simulink model "Auto_microgrid_forecasting_021622"  (R2020a)
settings: Solver=VariableStepAuto  StartTime=0.0  StopTime=50  MaxStep=1e-4  RelTol=1e-3
PreLoadFcn:
  | %run('FC_microgrid_param.m')
  | %load('gen_grid_init.mat')
InitFcn:
  | %load myisoModel_init;
  | run('FC_microgrid_param.m')
  | tic
  | run('CARTinitFcn.m')
  | %caseNo = 2;
  | 
  | %if (caseNo == 1)
  | %set_param(['Isolated_grid_paper_model_022521/SignalGen'], 'ActiveScenario', 'PStep222kW');
  | %else
  | %set_param(['Isolated_grid_paper_model_022521/SignalGen'], 'ActiveScenario', 'QStep222kVAr');
  | 
  | %end;
StopFcn:
  | toc
undefined symbols (not defined in the file or in its folder): breakpoints1, breakpoints2, cc_kp, cp_table_data, ctrl, D1, Delta, DiscIntNeverNeededParam, DT, FC_BESS, FC_PV_FirstSolar, find_system, Fnom, gcbh, libFC_BESS, libFC_PV, LowerLimit, magnitude, oversize, pll_ki, pll_kp, pq_ts, SOC_target, sps_rtmsupport, timer, Ts, ts, Ts_APC, Ts_Control, Ts_Power, UpperLimit
libraries: powerlib x151, simulink x100, powerlib_extras x100, powerlib_meascontrol x91, eePowerMeasurement x26, pi_ctrl x16, simulink_extras x12, sps_avr x7, eeGeneralControl x5, spsDieselMotorModel x3, libFSArray x2, SignalEditorBlockLib x2
(part 7 of 14)

== system Auto_microgrid_forecasting_021622/Grid Feeder Protective Relay/CS Modified PLL1/VCO ==
  w : Inport
  Compare To Constant : simulink/Logic and Bit Operations/Compare To Constant  relop=>=  const=pi  OutDataTypeStr=uint8
  Gain : Gain  Gain=2*pi  OutDataTypeStr=double
  Gain2 : Gain  Gain=Ts  SaturateOnIntegerOverflow=on  OutDataTypeStr=Inherit: Same as input  ParamDataTypeStr=Inherit: Same as input
  Sum : Sum  Inputs=-++
  Unit Delay1 : UnitDelay  SampleTime=-1  HasFrameUpgradeWarning=on
  theta : Outport
  wires:
  w/1 -> Gain2/1
  Gain/1 -> Sum/1
  Compare To Constant/1 -> Gain/1
  Unit Delay1/1 -> Compare To Constant/1, Sum/3, theta/1  "wt"
  Gain2/1 -> Sum/2
  Sum/1 -> Unit Delay1/1

== system Auto_microgrid_forecasting_021622/Grid Feeder Protective Relay/R25 - Sync Check v0.1/Freq_Comparator ==
  note: This block compares the frequency at the circuit breaker terminals
      | * if the difference is less than threshold dF_threshold, then outputs 1
  f_grid : Inport
  f_gen : Inport  Port=2
  dF_threshold : Inport  Port=3
  Fcn2 : Fcn  Expr=abs(u(2)-u(1)) <= u(3)
  Mux1 : Mux  Inputs=3
  Sum : Sum  Inputs=+-
  Locked : Outport
  dF : Outport  Port=2
  wires:
  Sum/1 -> dF/1
  f_grid/1 -> Mux1/1, Sum/2
  f_gen/1 -> Mux1/2, Sum/1
  dF_threshold/1 -> Mux1/3
  Fcn2/1 -> Locked/1
  Mux1/1 -> Fcn2/1

== system Auto_microgrid_forecasting_021622/Grid Feeder Protective Relay/R25 - Sync Check v0.1/Phase_Comparator ==
  note: This block compares the angle (phase A only) at the circuit breaker terminals
      | * if the difference is less than threshold angle_threshold, then outputs 1
  wt_grid : Inport
  wt_gen : Inport  Port=2
  angle_threshold : Inport  Port=3
  Abs : Abs
  Fcn1 : Fcn  Expr=u(1) <= u(2)  SampleTime=Ts
  Mux1 : Mux  Inputs=2
  Radians to Degrees : simulink_extras/Transformations/Radians to Degrees
  Scope : Scope
  Sum1 : Sum  Inputs=|-+
  WrapPi : Subsystem
  Locked : Outport
  dWt : Outport  Port=2
  wires:
  WrapPi/1(Out1) -> Abs/1, dWt/1
  Sum1/1 -> WrapPi/1(In1)
  wt_grid/1 -> Sum1/1
  wt_gen/1 -> Sum1/2
  Radians to Degrees/1 -> Scope/1, Mux1/1  "R2D"
  Mux1/1 -> Fcn1/1
  angle_threshold/1 -> Mux1/2
  Fcn1/1 -> Locked/1  "bool"
  Abs/1 -> Radians to Degrees/1  "diff"

== system Auto_microgrid_forecasting_021622/Grid Feeder Protective Relay/R25 - Sync Check v0.1/Voltage_Comparator ==
  note: This block compares the voltage at the circuit breaker terminals
      | * if the difference is less than threshold, then outputs 1
  note: dV_threshold% of the nominal VRMSLL
  V_bus : Inport
  V_line : Inport  Port=2
  dV_threshold : Inport  Port=3
  Fcn2 : Fcn  Expr=abs(u(2)-u(1)) <= u(3)
  Mux1 : Mux  Inputs=3
  Sum : Sum  Inputs=+-
  Locked : Outport
  dV : Outport  Port=2
  wires:
  Sum/1 -> dV/1
  dV_threshold/1 -> Mux1/3  "[%]"
  V_bus/1 -> Sum/2, Mux1/1
  V_line/1 -> Mux1/2, Sum/1
  Fcn2/1 -> Locked/1  "thshld"
  Mux1/1 -> Fcn2/1

== system Auto_microgrid_forecasting_021622/Grid Feeder Protective Relay1/CS Modified PLL/Controller ==
  note: Discrete PID Controller
  note: Pierre Giroux, Gilbert Sybille
      | Power System Simulation Laboratory
      | IREQ, Hydro-Quebc
  Error : Inport
  Discrete Derivative : simulink/Discrete/Discrete Derivative  gainval=1.0  ICPrevScaledInput=0.0  OutMin=[]  OutMax=[]  OutDataType=sfix(16)  OutScaling=2^-10  DoSatur=off
  Discrete-Time Integrator : DiscreteIntegrator  InitialCondition=Init  SampleTime=Ts  LimitOutput=on  UpperSaturationLimit=UpperLimit  LowerSaturationLimit=LowerLimit  ICPrevOutput=DiscIntNeverNeededParam  ICPrevScaledInput=DiscIntNeverNeededParam
  Kp4 : Gain  Gain=Kp  SaturateOnIntegerOverflow=on  OutDataTypeStr=Inherit: Same as input  ParamDataTypeStr=Inherit: Same as input
  Kp5 : Gain  Gain=Ki  SaturateOnIntegerOverflow=on  OutDataTypeStr=Inherit: Same as input  ParamDataTypeStr=Inherit: Same as input
  Kp6 : Gain  Gain=Kd  SaturateOnIntegerOverflow=on  OutDataTypeStr=Inherit: Same as input  ParamDataTypeStr=Inherit: Same as input
  Saturation2 : Saturate  UpperLimit=UpperLimit  LowerLimit=LowerLimit
  Sum6 : Sum  Inputs=+++  InputSameDT=on  SaturateOnIntegerOverflow=on  OutDataTypeStr=Inherit: Same as first input
  Zero-Order Hold : ZeroOrderHold  SampleTime=Ts
  Out : Outport  InitialOutput=0
  wires:
  Zero-Order Hold/1 -> Discrete Derivative/1
  Saturation2/1 -> Out/1
  Discrete Derivative/1 -> Sum6/3
  Discrete-Time Integrator/1 -> Sum6/2
  Kp4/1 -> Sum6/1
  Kp6/1 -> Zero-Order Hold/1
  Kp5/1 -> Discrete-Time Integrator/1
  Sum6/1 -> Saturation2/1
  Error/1 -> Kp6/1, Kp5/1, Kp4/1

== system Auto_microgrid_forecasting_021622/Grid Feeder Protective Relay1/CS Modified PLL/VCO ==
  w : Inport
  Compare To Constant : simulink/Logic and Bit Operations/Compare To Constant  relop=>=  const=pi  OutDataTypeStr=uint8
  Gain : Gain  Gain=2*pi  OutDataTypeStr=double
  Gain2 : Gain  Gain=Ts  SaturateOnIntegerOverflow=on  OutDataTypeStr=Inherit: Same as input  ParamDataTypeStr=Inherit: Same as input
  Sum : Sum  Inputs=-++
  Unit Delay1 : UnitDelay  SampleTime=-1  HasFrameUpgradeWarning=on
  theta : Outport
  wires:
  Sum/1 -> Unit Delay1/1
  Gain2/1 -> Sum/2
  Unit Delay1/1 -> theta/1, Sum/3, Compare To Constant/1  "wt"
  Compare To Constant/1 -> Gain/1
  Gain/1 -> Sum/1
  w/1 -> Gain2/1

== system Auto_microgrid_forecasting_021622/Grid Feeder Protective Relay1/CS Modified PLL1/Controller ==
  note: Discrete PID Controller
  note: Pierre Giroux, Gilbert Sybille
      | Power System Simulation Laboratory
      | IREQ, Hydro-Quebc
  Error : Inport
  Discrete Derivative : simulink/Discrete/Discrete Derivative  gainval=1.0  ICPrevScaledInput=0.0  OutMin=[]  OutMax=[]  OutDataType=sfix(16)  OutScaling=2^-10  DoSatur=off
  Discrete-Time Integrator : DiscreteIntegrator  InitialCondition=Init  SampleTime=Ts  LimitOutput=on  UpperSaturationLimit=UpperLimit  LowerSaturationLimit=LowerLimit  ICPrevOutput=DiscIntNeverNeededParam  ICPrevScaledInput=DiscIntNeverNeededParam
  Kp4 : Gain  Gain=Kp  SaturateOnIntegerOverflow=on  OutDataTypeStr=Inherit: Same as input  ParamDataTypeStr=Inherit: Same as input
  Kp5 : Gain  Gain=Ki  SaturateOnIntegerOverflow=on  OutDataTypeStr=Inherit: Same as input  ParamDataTypeStr=Inherit: Same as input
  Kp6 : Gain  Gain=Kd  SaturateOnIntegerOverflow=on  OutDataTypeStr=Inherit: Same as input  ParamDataTypeStr=Inherit: Same as input
  Saturation2 : Saturate  UpperLimit=UpperLimit  LowerLimit=LowerLimit
  Sum6 : Sum  Inputs=+++  InputSameDT=on  SaturateOnIntegerOverflow=on  OutDataTypeStr=Inherit: Same as first input
  Zero-Order Hold : ZeroOrderHold  SampleTime=Ts
  Out : Outport  InitialOutput=0
  wires:
  Zero-Order Hold/1 -> Discrete Derivative/1
  Saturation2/1 -> Out/1
  Discrete Derivative/1 -> Sum6/3
  Discrete-Time Integrator/1 -> Sum6/2
  Kp4/1 -> Sum6/1
  Kp6/1 -> Zero-Order Hold/1
  Kp5/1 -> Discrete-Time Integrator/1
  Sum6/1 -> Saturation2/1
  Error/1 -> Kp6/1, Kp5/1, Kp4/1

== system Auto_microgrid_forecasting_021622/Grid Feeder Protective Relay1/CS Modified PLL1/VCO ==
  w : Inport
  Compare To Constant : simulink/Logic and Bit Operations/Compare To Constant  relop=>=  const=pi  OutDataTypeStr=uint8
  Gain : Gain  Gain=2*pi  OutDataTypeStr=double
  Gain2 : Gain  Gain=Ts  SaturateOnIntegerOverflow=on  OutDataTypeStr=Inherit: Same as input  ParamDataTypeStr=Inherit: Same as input
  Sum : Sum  Inputs=-++
  Unit Delay1 : UnitDelay  SampleTime=-1  HasFrameUpgradeWarning=on
  theta : Outport
  wires:
  Sum/1 -> Unit Delay1/1
  Gain2/1 -> Sum/2
  Unit Delay1/1 -> theta/1, Sum/3, Compare To Constant/1  "wt"
  Compare To Constant/1 -> Gain/1
  Gain/1 -> Sum/1
  w/1 -> Gain2/1

== system Auto_microgrid_forecasting_021622/Grid Feeder Protective Relay1/R25 - Sync Check v0.1/Freq_Comparator ==
  note: This block compares the frequency at the circuit breaker terminals
      | * if the difference is less than threshold dF_threshold, then outputs 1
  f_grid : Inport
  f_gen : Inport  Port=2
  dF_threshold : Inport  Port=3
  Fcn2 : Fcn  Expr=abs(u(2)-u(1)) <= u(3)
  Mux1 : Mux  Inputs=3
  Sum : Sum  Inputs=+-
  Locked : Outport
  dF : Outport  Port=2
  wires:
  Mux1/1 -> Fcn2/1
  Fcn2/1 -> Locked/1
  dF_threshold/1 -> Mux1/3
  f_gen/1 -> Sum/1, Mux1/2
  f_grid/1 -> Sum/2, Mux1/1
  Sum/1 -> dF/1

== system Auto_microgrid_forecasting_021622/Grid Feeder Protective Relay1/R25 - Sync Check v0.1/Phase_Comparator ==
  note: This block compares the angle (phase A only) at the circuit breaker terminals
      | * if the difference is less than threshold angle_threshold, then outputs 1
  wt_grid : Inport
  wt_gen : Inport  Port=2
  angle_threshold : Inport  Port=3
  Abs : Abs
  Fcn1 : Fcn  Expr=u(1) <= u(2)  SampleTime=Ts
  Mux1 : Mux  Inputs=2
  Radians to Degrees : simulink_extras/Transformations/Radians to Degrees
  Scope : Scope
  Sum1 : Sum  Inputs=|-+
  WrapPi : Subsystem
  Locked : Outport
  dWt : Outport  Port=2
  wires:
  Abs/1 -> Radians to Degrees/1  "diff"
  Fcn1/1 -> Locked/1  "bool"
  angle_threshold/1 -> Mux1/2
  Mux1/1 -> Fcn1/1
  Radians to Degrees/1 -> Scope/1, Mux1/1  "R2D"
  wt_gen/1 -> Sum1/2
  wt_grid/1 -> Sum1/1
  Sum1/1 -> WrapPi/1(In1)
  WrapPi/1(Out1) -> dWt/1, Abs/1

== system Auto_microgrid_forecasting_021622/Grid Feeder Protective Relay1/R25 - Sync Check v0.1/Voltage_Comparator ==
  note: dV_threshold% of the nominal VRMSLL
  note: This block compares the voltage at the circuit breaker terminals
      | * if the difference is less than threshold, then outputs 1
  V_bus : Inport
  V_line : Inport  Port=2
  dV_threshold : Inport  Port=3
  Fcn2 : Fcn  Expr=abs(u(2)-u(1)) <= u(3)
  Mux1 : Mux  Inputs=3
  Sum : Sum  Inputs=+-
  Locked : Outport
  dV : Outport  Port=2
  wires:
  Mux1/1 -> Fcn2/1
  Fcn2/1 -> Locked/1  "thshld"
  V_line/1 -> Sum/1, Mux1/2
  V_bus/1 -> Mux1/1, Sum/2
  dV_threshold/1 -> Mux1/3  "[%]"
  Sum/1 -> dV/1

== system Auto_microgrid_forecasting_021622/MODEL STABILIZER/AllStringInverters/BESS Inverter ==
  ctrl : Inport
  Controlled Voltage Source : powerlib/Electrical Sources/Controlled Voltage Source  Initialize=on  Source_Type=AC  Amplitude=0  Phase=0  Frequency=0  Measurements=None
  Controlled Voltage Source1 : powerlib/Electrical Sources/Controlled Voltage Source  Initialize=on  Source_Type=AC  Amplitude=0  Phase=0  Frequency=0  Measurements=None
  Controlled Voltage Source2 : powerlib/Electrical Sources/Controlled Voltage Source  Initialize=on  Source_Type=AC  Amplitude=0  Phase=0  Frequency=0  Measurements=None
  Demux : Demux  Outputs=3
  A : PMIOPort  Side=Right
  N : PMIOPort  Port=2  Side=Left
  B : PMIOPort  Port=3  Side=Right
  C : PMIOPort  Port=4  Side=Right
  wires:
  Demux/1 -> Controlled Voltage Source/1
  Demux/2 -> Controlled Voltage Source1/1
  Demux/3 -> Controlled Voltage Source2/1
  ctrl/1 -> Demux/1
  connections:
  A/RConn1 -- Controlled Voltage Source/RConn1
  Controlled Voltage Source2/LConn1 -- Controlled Voltage Source/LConn1 -- Controlled Voltage Source1/LConn1 -- N/RConn1
  Controlled Voltage Source1/RConn1 -- B/RConn1
  Controlled Voltage Source2/RConn1 -- C/RConn1

== system Auto_microgrid_forecasting_021622/MODEL STABILIZER/AllStringInverters/Stab_control ==
  Uabc : Inport
  Uabc_inv : Inport  Port=2
  Iabc : Inport  Port=3
  CB_status : Inport  Port=4
  Control : Inport  Port=5
  Bus Creator1 : BusCreator  Inputs=2
  Bus Creator5 : BusCreator  Inputs=1
  Bus Selector : BusSelector  OutputSignals=p_ref,q_ref,f_ref,v_ref,GF_mode
  InvControl : Subsystem  mask{Ts=Ts_Control, Unpp=600, Pn=200e3}
      mask prompts: Ts "Control sample time [s]"; Unpp "Nominal AC voltage [Vpp]"; Pn "Nominal Power [W]"
      mask init:
      | Unom = Unpp / sqrt(3);
      | Inom = Pn/3/Unom;
  Rate Transition{,1..2,4..7,9..10} (9 alike) : RateTransition  Integrity=off  OutPortSampleTime=Ts_Control
  Rate Transition3 : RateTransition  OutPortSampleTime=Ts
  Rate Transition8 : RateTransition  OutPortSampleTime=Ts
  Step1 : Step  Time=99  SampleTime=0
  Step2 : Step  Time=100  After=-1  SampleTime=0
  Sum : Sum  Inputs=|++
  CtrlOut : Outport
  wires:
  Sum/1 -> Rate Transition8/1
  Rate Transition10/1 -> InvControl/2(Uabc_inv)
  Uabc_inv/1 -> Rate Transition10/1
  Control/1 -> Bus Selector/1
  Rate Transition6/1 -> InvControl/7(fref)
  Rate Transition5/1 -> InvControl/6(qref)
  Rate Transition7/1 -> InvControl/8(vref)
  Rate Transition9/1 -> InvControl/9(GF_mode_en)
  Bus Selector/5 -> Rate Transition9/1  "<GF_mode>"
  Bus Selector/4 -> Rate Transition7/1  "<v_ref>"
  Bus Selector/3 -> Rate Transition6/1  "<f_ref>"
  Bus Selector/2 -> Rate Transition5/1  "<q_ref>"
  Bus Selector/1 -> Rate Transition4/1  "<p_ref>"
  Bus Creator1/1 -> CtrlOut/1
  Bus Creator5/1 -> Bus Creator1/2  "ToCB"
  CB_status/1 -> Rate Transition2/1
  Uabc/1 -> Rate Transition/1
  Rate Transition3/1 -> Bus Creator1/1  "Uabc"
  InvControl/1(Uabc_ref) -> Rate Transition3/1
  Rate Transition8/1 -> Bus Creator5/1  "Close"
  Rate Transition/1 -> InvControl/1(Uabc)
  Rate Transition1/1 -> InvControl/3(Iabc)
  Rate Transition2/1 -> InvControl/4(cb_stat)
  Iabc/1 -> Rate Transition1/1
  Rate Transition4/1 -> InvControl/5(pref)
  Step1/1 -> Sum/1
  Step2/1 -> Sum/2

== system Auto_microgrid_forecasting_021622/MODEL STABILIZER/AllStringInverters/Subsystem1 ==
  SmaINV : powerlib/Measurements/Three-Phase V-I Measurement  VoltageMeasurement=phase-to-ground  SetLabelV=off  LabelV=circuit_Usmainv  Vpu=off  VpuLL=off  CurrentMeasurement=yes  SetLabelI=off  LabelI=circuit_Ismainv  Ipu=off  Pbase=100e6  Vbase=500e3  OutputType=Complex  PhasorSimulation=off  PSBequivalent=0
  A : PMIOPort  Side=Left
  a : PMIOPort  Port=2  Side=Right
  B : PMIOPort  Port=3  Side=Left
  b : PMIOPort  Port=4  Side=Right
  C : PMIOPort  Port=5  Side=Left
  c : PMIOPort  Port=6  Side=Right
  tag scope: Iinv=scoped, Uinv=scoped
  wires:
  SmaINV/1 -> [Uinv]
  SmaINV/2 -> [Iinv]
  connections:
  SmaINV/RConn1 -- a/RConn1
  C/RConn1 -- SmaINV/LConn3
  SmaINV/LConn2 -- B/RConn1
  SmaINV/RConn2 -- b/RConn1
  SmaINV/RConn3 -- c/RConn1
  A/RConn1 -- SmaINV/LConn1

== system Auto_microgrid_forecasting_021622/MODEL STABILIZER/AllStringInverters/Subsystem2 ==
  GRI1 : powerlib/Measurements/Three-Phase V-I Measurement  VoltageMeasurement=phase-to-ground  SetLabelV=off  LabelV=Ugri  Vpu=off  VpuLL=off  CurrentMeasurement=yes  SetLabelI=off  LabelI=Igri  Ipu=off  Pbase=100e6  Vbase=500e3  OutputType=Complex  PhasorSimulation=off  PSBequivalent=0
  A : PMIOPort  Side=Left
  B : PMIOPort  Port=2  Side=Left
  a : PMIOPort  Port=3  Side=Right
  b : PMIOPort  Port=4  Side=Right
  C : PMIOPort  Port=5  Side=Left
  c : PMIOPort  Port=6  Side=Right
  tag scope: Igri=scoped, Ugri=scoped
  wires:
  GRI1/1 -> [Ugri]
  GRI1/2 -> [Igri]
  connections:
  GRI1/LConn3 -- C/RConn1
  GRI1/LConn2 -- B/RConn1
  GRI1/RConn3 -- c/RConn1
  GRI1/RConn2 -- b/RConn1
  GRI1/LConn1 -- A/RConn1
  GRI1/RConn1 -- a/RConn1

== system Auto_microgrid_forecasting_021622/Stab1/AllStringInverters/BESS Inverter ==
  ctrl : Inport
  Controlled Voltage Source : powerlib/Electrical Sources/Controlled Voltage Source  Initialize=on  Source_Type=AC  Amplitude=0  Phase=0  Frequency=0  Measurements=None
  Controlled Voltage Source1 : powerlib/Electrical Sources/Controlled Voltage Source  Initialize=on  Source_Type=AC  Amplitude=0  Phase=0  Frequency=0  Measurements=None
  Controlled Voltage Source2 : powerlib/Electrical Sources/Controlled Voltage Source  Initialize=on  Source_Type=AC  Amplitude=0  Phase=0  Frequency=0  Measurements=None
  Demux : Demux  Outputs=3
  A : PMIOPort  Side=Right
  N : PMIOPort  Port=2  Side=Left
  B : PMIOPort  Port=3  Side=Right
  C : PMIOPort  Port=4  Side=Right
  wires:
  ctrl/1 -> Demux/1
  Demux/3 -> Controlled Voltage Source2/1
  Demux/2 -> Controlled Voltage Source1/1
  Demux/1 -> Controlled Voltage Source/1
  connections:
  Controlled Voltage Source2/RConn1 -- C/RConn1
  Controlled Voltage Source1/RConn1 -- B/RConn1
  N/RConn1 -- Controlled Voltage Source1/LConn1 -- Controlled Voltage Source/LConn1 -- Controlled Voltage Source2/LConn1
  A/RConn1 -- Controlled Voltage Source/RConn1

== system Auto_microgrid_forecasting_021622/Stab1/AllStringInverters/PV_Control ==
  Uabc : Inport
  Uabc_inv : Inport  Port=2
  Iabc : Inport  Port=3
  CB_status : Inport  Port=4
  Control : Inport  Port=5
  Bus Creator1 : BusCreator  Inputs=2
  Bus Creator5 : BusCreator  Inputs=1
  Bus Selector : BusSelector  OutputSignals=p_ref,q_ref,f_ref,v_ref,GF_mode
  InvControl : Subsystem  mask{Ts=Ts_Control, Unpp=600, Pn=430e3}
      mask prompts: Ts "Control sample time [s]"; Unpp "Nominal AC voltage [Vpp]"; Pn "Nominal Power [W]"
      mask init:
      | Unom = Unpp / sqrt(3);
      | Inom = Pn/3/Unom;
  Rate Transition{,1..2,4..7,9..10} (9 alike) : RateTransition  Integrity=off  OutPortSampleTime=Ts_Control
  Rate Transition3 : RateTransition  OutPortSampleTime=Ts
  Rate Transition8 : RateTransition  OutPortSampleTime=Ts
  Step : Step  Time=3  SampleTime=0
  Step1 : Step  Time=6.4  SampleTime=0
  Sum : Sum  Inputs=|++
  CtrlOut : Outport
  wires:
  Step1/1 -> Sum/2
  Step/1 -> Sum/1
  Rate Transition4/1 -> InvControl/5(pref)
  Iabc/1 -> Rate Transition1/1
  Rate Transition2/1 -> InvControl/4(cb_stat)
  Rate Transition1/1 -> InvControl/3(Iabc)
  Rate Transition/1 -> InvControl/1(Uabc)
  Rate Transition8/1 -> Bus Creator5/1  "Close"
  Sum/1 -> Rate Transition8/1
  InvControl/1(Uabc_ref) -> Rate Transition3/1
  Rate Transition3/1 -> Bus Creator1/1  "Uabc"
  Uabc/1 -> Rate Transition/1
  CB_status/1 -> Rate Transition2/1
  Bus Creator5/1 -> Bus Creator1/2  "ToCB"
  Bus Creator1/1 -> CtrlOut/1
  Bus Selector/1 -> Rate Transition4/1  "<p_ref>"
  Bus Selector/2 -> Rate Transition5/1  "<q_ref>"
  Bus Selector/3 -> Rate Transition6/1  "<f_ref>"
  Bus Selector/4 -> Rate Transition7/1  "<v_ref>"
  Bus Selector/5 -> Rate Transition9/1  "<GF_mode>"
  Rate Transition9/1 -> InvControl/9(GF_mode_en)
  Rate Transition7/1 -> InvControl/8(vref)
  Rate Transition5/1 -> InvControl/6(qref)
  Rate Transition6/1 -> InvControl/7(fref)
  Control/1 -> Bus Selector/1
  Uabc_inv/1 -> Rate Transition10/1
  Rate Transition10/1 -> InvControl/2(Uabc_inv)

== system Auto_microgrid_forecasting_021622/Stab1/AllStringInverters/Subsystem1 ==
  SmaINV : powerlib/Measurements/Three-Phase V-I Measurement  VoltageMeasurement=phase-to-ground  SetLabelV=off  LabelV=circuit_Usmainv  Vpu=off  VpuLL=off  CurrentMeasurement=yes  SetLabelI=off  LabelI=circuit_Ismainv  Ipu=off  Pbase=100e6  Vbase=500e3  OutputType=Complex  PhasorSimulation=off  PSBequivalent=0
  A : PMIOPort  Side=Left
  a : PMIOPort  Port=2  Side=Right
  B : PMIOPort  Port=3  Side=Left
  b : PMIOPort  Port=4  Side=Right
  C : PMIOPort  Port=5  Side=Left
  c : PMIOPort  Port=6  Side=Right
  tag scope: Iinv=scoped, Uinv=scoped
  wires:
  SmaINV/2 -> [Iinv]
  SmaINV/1 -> [Uinv]
  connections:
  A/RConn1 -- SmaINV/LConn1
  SmaINV/RConn3 -- c/RConn1
  SmaINV/RConn2 -- b/RConn1
  SmaINV/LConn2 -- B/RConn1
  C/RConn1 -- SmaINV/LConn3
  SmaINV/RConn1 -- a/RConn1

== system Auto_microgrid_forecasting_021622/Stab1/AllStringInverters/Subsystem2 ==
  GRI1 : powerlib/Measurements/Three-Phase V-I Measurement  VoltageMeasurement=phase-to-ground  SetLabelV=off  LabelV=Ugri  Vpu=off  VpuLL=off  CurrentMeasurement=yes  SetLabelI=off  LabelI=Igri  Ipu=off  Pbase=100e6  Vbase=500e3  OutputType=Complex  PhasorSimulation=off  PSBequivalent=0
  A : PMIOPort  Side=Left
  B : PMIOPort  Port=2  Side=Left
  a : PMIOPort  Port=3  Side=Right
  b : PMIOPort  Port=4  Side=Right
  C : PMIOPort  Port=5  Side=Left
  c : PMIOPort  Port=6  Side=Right
  tag scope: Igri=scoped, Ugri=scoped
  wires:
  GRI1/2 -> [Igri]
  GRI1/1 -> [Ugri]
  connections:
  GRI1/RConn1 -- a/RConn1
  GRI1/LConn1 -- A/RConn1
  GRI1/RConn2 -- b/RConn1
  GRI1/RConn3 -- c/RConn1
  GRI1/LConn2 -- B/RConn1
  GRI1/LConn3 -- C/RConn1

== system Auto_microgrid_forecasting_021622/Wind Turbine Type 4/APC (atomic)1/Baseline ==
  Action Port : ActionPort  ActionPortLabel=case [ 5 ]:
  Constant1 : Constant  Value=0
  Qcmd : Outport
  dP : Outport  Port=2
  dT : Outport  Port=3
  wires:
  Constant1/1 -> dP/1, dT/1, Qcmd/1

== system Auto_microgrid_forecasting_021622/Wind Turbine Type 4/APC (atomic)1/Inertial Response (to df) ==
  Freq (Hz) : Inport
  type1 : Inport  Port=2
  wg (pu) : Inport  Port=3
  f_setpoint : Inport  Port=4
  Action Port : ActionPort  ActionPortLabel=case [ 1 ]:
  Constant1 : Constant  Value=0
  Constant2 : Constant  Value=0
  Constant3 : Constant  Value=1e-3
  Display{3..4,6..7} (4 alike) : Display
  Divide1 : Product  Inputs=*/
  FBIC : Subsystem
  Gain : Gain  Gain=Fnom
  Lock2 : Subsystem
  Rate Limiter1 : RateLimiter  RisingSlewLimit=0.45  SampleTimeMode=inherited
  Relational Operator3 : RelationalOperator  OutDataTypeStr=boolean  RndMeth=Nearest
  Relational Operator4 : RelationalOperator  Operator=<=  OutDataTypeStr=boolean  RndMeth=Nearest
  Saturation : Saturate  UpperLimit=0.4  LowerLimit=0
  Saturation1 : Saturate  UpperLimit=1  LowerLimit=1e-5
  Scope : Scope  NumInputPorts=3
  Sum1 : Sum  Inputs=|-+
  Switch1 : Switch  Criteria=u2 > Threshold  Threshold=1
  TLIC : Subsystem  TreatAsAtomicUnit=on
  Type1 : Switch  Criteria=u2 > Threshold  Threshold=0.5
  When to start IR : DigitalClock  SampleTime=-1
  dead band1 : Constant  Value=0.2
  dT : Outport
  dP : Outport  Port=2
  Qcmd : Outport  Port=3
  wires:
  Constant1/1 -> dP/1, Qcmd/1
  Constant2/1 -> Switch1/3
  When to start IR/1 -> Switch1/2
  Lock2/1(O) -> Switch1/1
  Saturation/1 -> dT/1
  wg (pu)/1 -> [Wg], FBIC/1(wg (pu))
  Switch1/1 -> Display3/1, Scope/3, [In_Act]
  type1/1 -> Type1/2
  Sum1/1 -> Relational Operator3/1, Scope/2
  FBIC/1(Delta_P FBIC1) -> Type1/3
  Type1/1 -> [Delta_P], Display6/1
  Freq (Hz)/1 -> FBIC/2(Freq (Hz)1), [Freq]
  [In_Act] -> FBIC/3(Act1), TLIC/1(Act)
  TLIC/1(Delta_P TLIC) -> Type1/1
  [Delta_P] -> Relational Operator4/1
  f_setpoint/1 -> Gain/1
  dead band1/1 -> Relational Operator3/2
  Divide1/1 -> Rate Limiter1/1
  [Wg] -> Saturation1/1
  Saturation1/1 -> Divide1/2
  Constant3/1 -> Relational Operator4/2
  Relational Operator4/1 -> Display7/1, Lock2/2(R)
  [Freq] -> Sum1/1, Display4/1
  [Delta_P] -> Divide1/1, Scope/1
  Relational Operator3/1 -> Lock2/1(I)
  Rate Limiter1/1 -> Saturation/1
  Gain/1 -> Sum1/2

== system Auto_microgrid_forecasting_021622/Wind Turbine Type 4/APC (atomic)1/PFR ==
  Freq (Hz) : Inport
  f_setpoint : Inport  Port=2
  Action Port : ActionPort  ActionPortLabel=case [ 2 3 ]:
  Constant1 : Constant  Value=0
  Dead Zone : DeadZone  LowerValue=-db/60  UpperValue=db/60  SaturateOnIntegerOverflow=on
  Divide1 : Product  Inputs=*/
  Gain : Gain  Gain=Fnom
  P/f gain : Gain  Gain=1/k
  Saturation : Saturate  UpperLimit=0
  Sum : Sum  Inputs=|+-
  Sum1 : Sum  Inputs=|-+
  curtailment pu : Constant  Value=0.2
  dP : Outport
  dT : Outport  Port=2
  Qcmd : Outport  Port=3
  wires:
  Sum/1 -> Saturation/1
  Constant1/1 -> dT/1, Qcmd/1
  Saturation/1 -> dP/1
  P/f gain/1 -> Sum/1
  curtailment pu/1 -> Sum/2
  Dead Zone/1 -> P/f gain/1
  f_setpoint/1 -> Gain/1
  Freq (Hz)/1 -> Sum1/1
  Divide1/1 -> Dead Zone/1  "delta f pu"
  Sum1/1 -> Divide1/1
  Gain/1 -> Sum1/2, Divide1/2

== system Auto_microgrid_forecasting_021622/Wind Turbine Type 4/APC (atomic)1/PQ ==
  SFRcmd : Inport
  Qin : Inport  Port=2
  Action Port : ActionPort  ActionPortLabel=case [ 4 ]:
  Constant : Constant
  Constant1 : Constant  Value=0
  Sum : Sum  Inputs=|+-
  dP : Outport
  Qcmd : Outport  Port=2
  dT : Outport  Port=3
  wires:
  Constant1/1 -> dT/1
  Qin/1 -> Qcmd/1
  Constant/1 -> Sum/2
  Sum/1 -> dP/1
  SFRcmd/1 -> Sum/1

== system Auto_microgrid_forecasting_021622/Wind Turbine Type 4/Control/Excitation Control system ==
  Flux : Inport
  wr : Inport  Port=2
  Discrete PI Controller : Subsystem  DialogController=POWERSYS.PowerSysDialog  mask(Discrete PI Controller){Kp=Kp_field, Ki=Ki_field, Par_Limits=[1 0]*Vf_limit, Init=init(9), Ts=Ts}
      mask prompts: Kp "Proportional gain (Kp):"; Ki "Integral gain (Ki):"; Par_Limits "Output limits: [ Upper   Lower ]"; Init "Output initial value:"; Ts "Sample time:"
      mask help: This block implements a discrete PI controller.
      mask init:
      | UpperLimit=Par_Limits(1);
      | LowerLimit=Par_Limits(2);
      | power_initmask();
      mask Help: This block is part of a subset of blocks in the Extras library that does not have documentation associated with it, other than the block mask description.
      mask Display: disp('PI');
  Divide : Product  Inputs=*/
  Flux_ref : Constant
  "Flux_ref " : Constant
  Sum4 : Sum  Inputs=|+-  InputSameDT=on  SaturateOnIntegerOverflow=on  OutDataTypeStr=Inherit: Same as first input
  Switch : Switch  Threshold=1
  avoid division by 0 : Saturate  UpperLimit=inf  LowerLimit=1e-6
  Vf : Outport  VectorParamsAs1DForOutWhenUnconnected=off
  wires:
  Sum4/1 -> Discrete PI Controller/1(Error)
  Discrete PI Controller/1(Out) -> Vf/1  "Vf"
  Flux/1 -> Sum4/2  "Flux"
  wr/1 -> Switch/2, avoid division by 0/1
  Flux_ref/1 -> Switch/3
  "Flux_ref "/1 -> Divide/1
  avoid division by 0/1 -> Divide/2
  Divide/1 -> Switch/1
  Switch/1 -> Sum4/1

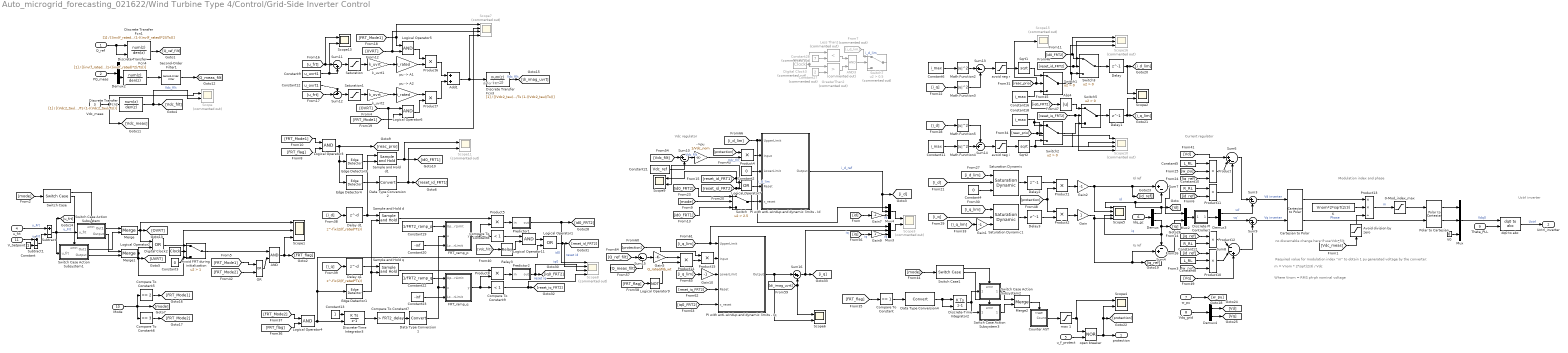
== system Auto_microgrid_forecasting_021622/Wind Turbine Type 4/Control/Grid-Side Inverter Control ==
  note: no discernable change here if use Vdc_filt
  note: di for FRT
  note: Required value for modulation index "m" to obtain 1 pu generated voltage by the converter:
  note: Modulation index and phase
  note: Where Vnom = RMS ph-ph nominal voltage
  note: Uctrl inverter
  note: Current regulator
  note: Iq ref
  note: m = Vnom * 2*sqrt(2/3) / Vdc
  note: Id ref
  note: Vdc regulator
  Q_ref : Inport
  PQ_meas : Inport  Port=2
  Vdc_meas : Inport  Port=3
  u_frt : Inport  Port=4
  u_f_protect : Inport  Port=5
  Idq_gc : Inport  Port=6
  w_pu : Inport  Port=7
  Vdq_grid : Inport  Port=8
  Theta_PLL : Inport  Port=9
  Mode : Inport  Port=10
  V_Setpoint : Inport  Port=11
  ->pu : Gain  Gain=1/Vdc_nom
  0-Mod_index_max : Saturate  UpperLimit=Mod_index_max  LowerLimit=0
  AND : Logic  IconShape=distinctive  AllPortsSameDT=off  OutDataTypeStr=boolean
  AND3 : Logic  Commented=on  IconShape=distinctive  AllPortsSameDT=off  OutDataTypeStr=boolean
  Abs4 : Abs
  Add1 : Sum
  Avoid FRT during initialization : Switch  Criteria=u2 > Threshold  Threshold=1
  Avoid division by zero : Saturate  UpperLimit=1e6  LowerLimit=1e-6
  Cartesian to Polar : simulink_extras/Transformations/Cartesian to Polar
  Compare To Constant : simulink/Logic and Bit Operations/Compare To Constant  relop===  const=1  OutDataTypeStr=boolean
  Compare To Constant5 : simulink/Logic and Bit Operations/Compare To Constant  relop===  const=2  OutDataTypeStr=boolean
  Compare To Constant6 : simulink/Logic and Bit Operations/Compare To Constant  relop===  const=3  OutDataTypeStr=boolean
  Compare To Constant7 : simulink/Logic and Bit Operations/Compare To Constant  relop=>  const=FRT2_delay  OutDataTypeStr=boolean
  Compare To Constant8 : simulink/Logic and Bit Operations/Compare To Constant  relop=<  const=1  OutDataTypeStr=boolean
  Compare To Constant9 : simulink/Logic and Bit Operations/Compare To Constant  relop=<  const=1  OutDataTypeStr=boolean
  Constant : Constant
  Constant10 : Constant  Value=R_RL
  Constant{6,11,16,18} (4 alike) : Constant  Value=i_max  SampleTime=Ts
  Constant12 : Constant  Value=u_ovrt1  SampleTime=Ts
  Constant13 : Constant
  Constant17 : Constant  Value=R_RL
  Constant19 : Constant  Value=1/FRT2_ramp_p  SampleTime=Ts
  Constant2 : Constant  Value=0  SampleTime=Ts
  Constant20 : Constant  Value=-inf  SampleTime=Ts
  Constant21 : Constant  Value=Vdc_ref  SampleTime=Ts
  Constant22 : Constant  Value=1/FRT2_ramp_q  SampleTime=Ts
  Constant23 : Constant  Value=-inf  SampleTime=Ts
  Constant27 : Constant  Commented=on  Value=2
  Constant28 : Constant  Commented=on  Value=7
  Constant3 : Constant  Value=0
  Constant4 : Constant  Value=0  SampleTime=Ts
  Constant5 : Constant  Value=L_RL
  Constant8 : Constant  Value=L_RL
  Constant9 : Constant  Value=u_uvrt1  SampleTime=Ts
  Counter AST : Subsystem
  Data Type Conversion1 : DataTypeConversion
  Data Type Conversion2 : DataTypeConversion
  Data Type Conversion4 : DataTypeConversion
  Delay{,1..3} (4 alike) : Delay  DelayLength=1  InitialCondition=0  SampleTime=Ts
  Delay d1 : Delay  DelayLength=fix(2/(f_rated*Ts))  InitialCondition=1  SampleTime=Ts
  Delay q1 : Delay  DelayLength=fix(2/(f_rated*Ts))  InitialCondition=1  SampleTime=Ts
  Demux{,2..4} (4 alike) : Demux  Outputs=2
      Demux settings: DisplayOption=none
      Demux3 settings: DisplayOption=none
      Demux4 settings: DisplayOption=none
  Digital Clock2 : DigitalClock  SampleTime=Ts
  Digital Clock3 : DigitalClock  Commented=on  SampleTime=-1
  Discrete PI Controller1 : Subsystem  DialogController=POWERSYS.PowerSysDialog  mask(Discrete PI Controller){Kp=Kp_grid_side_cur_reg, Ki=Ki_grid_side_cur_reg, Par_Limits=[1 -1]*Current_reg_output_limit, Init=0, Ts=Ts}
      mask prompts: Kp "Proportional gain (Kp):"; Ki "Integral gain (Ki):"; Par_Limits "Output limits: [ Upper   Lower ]"; Init "Output initial value:"; Ts "Sample time:"
      mask help: This block implements a discrete PI controller.
      mask init:
      | UpperLimit=Par_Limits(1);
      | LowerLimit=Par_Limits(2);
      | power_initmask();
      mask Help: This block is part of a subset of blocks in the Extras library that does not have documentation associated with it, other than the block mask description.
      mask Display: disp('PI');
  Discrete Transfer Fcn1 : DiscreteTransferFcn  Denominator=[(inv(f_rated)*2)/Ts (1-((inv(f_rated)*2)/Ts))]  InitialStatesSource=Input port  SampleTime=Ts
      settings: InputPortMap=u0,p5
  Discrete Transfer Fcn2 : DiscreteTransferFcn  Denominator=[(Vdc2_tau)/Ts (1-((Vdc2_tau)/Ts))]  InitialStates=Vdc2_filt_init  SampleTime=Ts
  Discrete Transfer Fcn3 : DiscreteTransferFcn  Denominator=[(Vdc2_tau)/Ts (1-((Vdc2_tau)/Ts))]  SampleTime=Ts
  Discrete Transfer Fcn4 : DiscreteTransferFcn  Denominator=[(inv(f_rated)*2)/Ts (1-((inv(f_rated)*2)/Ts))]  InitialStates=U_rated^2/(-inv(2*pi*f_rated*Cshunt_filter))  SampleTime=Ts
  Discrete-Time Integrator2 : DiscreteIntegrator  ExternalReset=falling  SampleTime=Ts  ICPrevOutput=DiscIntNeverNeededParam  ICPrevScaledInput=DiscIntNeverNeededParam
  Discrete-Time Integrator3 : DiscreteIntegrator  ExternalReset=level  SampleTime=Ts  LimitOutput=on  UpperSaturationLimit=1  LowerSaturationLimit=0  ICPrevOutput=DiscIntNeverNeededParam  ICPrevScaledInput=DiscIntNeverNeededParam
  Edge Detector1 : powerlib_meascontrol/Logic/Edge Detector  model=Rising  ic=0  Ts=Ts
      settings: SourceProductBaseCode=PS
  Edge Detector3 : powerlib_meascontrol/Logic/Edge Detector  model=Rising  ic=0  Ts=Ts
      settings: SourceProductBaseCode=PS
  Edge Detector4 : powerlib_meascontrol/Logic/Edge Detector  model=Falling  ic=0  Ts=Ts
      settings: SourceProductBaseCode=PS
  FRT_ramp_p : Subsystem
  FRT_ramp_q : Subsystem
  From7 : From  Commented=on  GotoTag=i_d_lim
  Gain : Gain
  Gain{1..2,7,10} (4 alike) : Gain  Gain=-1
  Gain5 : Gain  Gain=Q_rated/Nb_wt
  Gain9 : Gain
  GreaterThan2 : RelationalOperator  Commented=on  Operator=>  OutDataTypeStr=boolean  RndMeth=Simplest
  K : Constant  Value=Vnom*2*sqrt(2/3)
  Less Than2 : RelationalOperator  Commented=on  Operator=<  OutDataTypeStr=boolean  RndMeth=Simplest
  Logical Operator1 : Logic  Operator=OR  AllPortsSameDT=off  OutDataTypeStr=boolean
  Logical Operator{3..6,11} (5 alike) : Logic  AllPortsSameDT=off  OutDataTypeStr=boolean
  Logical Operator2 : Logic  Operator=OR  AllPortsSameDT=off  OutDataTypeStr=boolean
  Logical Operator7 : Logic  Operator=OR  AllPortsSameDT=off  OutDataTypeStr=boolean
  Logical Operator9 : Logic  Operator=NOT  AllPortsSameDT=off  OutDataTypeStr=boolean
  Math Function{2..5} (4 alike) : Math  Operator=magnitude^2  SignedPower=on  SaturateOnIntegerOverflow=on
  Merge : Merge
  Merge1 : Merge
  Merge2 : Merge
  Mux : Mux  Inputs=3
  Mux2 : Mux  Inputs=2
  Mux3 : Mux  Inputs=3
  Mux4 : Mux  Inputs=3
  OR : Logic  Operator=OR  IconShape=distinctive  AllPortsSameDT=off  OutDataTypeStr=boolean
  PI with anti-windup and dynamic limits - Id : Subsystem  mask(Discrete PI Controller with anti-windup and dynamic limiters){Kp=Kp_dc, Ki=Ki_dc, Init=Vdc_nom, Ts=Ts}
      mask prompts: Kp "Proportional gain (Kp):"; Ki "Integral gain (Ki):"; Init "State initial value:"; Ts "Sample time:"
      mask Display:
      | disp('PI-\nAST');
      | port_label('input',1,'Max');
      | port_label('input',2,'In');
      | port_label('input',3,'Min');
      | port_label('input',4,'Reset');
      | port_label('input',5,'x_reset');
      | port_label('output',1,'Out');
  PI with anti-windup and dynamic limits - Iq : Subsystem  mask(Discrete PI Controller with anti-windup and dynamic limiters){Kp=Q_Kp/1000, Ki=Q_Ki/1000, Init=0, Ts=Ts}
      mask prompts: Kp "Proportional gain (Kp):"; Ki "Integral gain (Ki):"; Init "State initial value:"; Ts "Sample time:"
      mask Display:
      | disp('PI-\nAST');
      | port_label('input',1,'Max');
      | port_label('input',2,'In');
      | port_label('input',3,'Min');
      | port_label('input',4,'Reset');
      | port_label('input',5,'x_reset');
      | port_label('output',1,'Out');
  Polar to Cartesian : simulink_extras/Transformations/Polar to Cartesian
      settings: SourceProductBaseCode=SL
  Predictor1 : Subsystem  mask{Init_value=0, Ts=Ts}
      mask prompts: Init_value "Initial value:"; Ts "Sample time (Ts):"
  Predictor2 : Subsystem  mask{Init_value=0, Ts=Ts}
      mask prompts: Init_value "Initial value:"; Ts "Sample time (Ts):"
  Product : Product  Inputs=3  InputSameDT=on  SaturateOnIntegerOverflow=on  OutDataTypeStr=Inherit: Same as first input
  Product{1..2,4..8,14..15} (9 alike) : Product
  Product10 : Product  Inputs=3  InputSameDT=on  SaturateOnIntegerOverflow=on  OutDataTypeStr=Inherit: Same as first input
  Product11 : Product  InputSameDT=on  SaturateOnIntegerOverflow=on  OutDataTypeStr=Inherit: Same as first input
  Product12 : Product  InputSameDT=on  SaturateOnIntegerOverflow=on  OutDataTypeStr=Inherit: Same as first input
  Product13 : Product  Inputs=**/  InputSameDT=on  SaturateOnIntegerOverflow=on  OutDataTypeStr=Inherit: Same as first input
  Relay3 : Relay  OnSwitchValue=1.02*Vdc_ref  OffSwitchValue=1.015*Vdc_ref  OutDataTypeStr=Inherit: Inherit via back propagation
  Sample and Hold d : powerlib_meascontrol/Additional Components/Sample and Hold  ic=0  Ts=Ts
      settings: SourceProductBaseCode=PS
  Sample and Hold d1 : powerlib_meascontrol/Additional Components/Sample and Hold  ic=0  Ts=Ts
      settings: SourceProductBaseCode=PS
  Sample and Hold q : powerlib_meascontrol/Additional Components/Sample and Hold  ic=0  Ts=Ts
      settings: SourceProductBaseCode=PS
  Saturation : Saturate  UpperLimit=0.08  LowerLimit=0
  Saturation Dynamic : simulink/Discontinuities/Saturation Dynamic  OutMin=[]  OutMax=[]  OutDataTypeStr=Inherit: Same as second input  OutDataType=fixdt(1, 16)  OutScaling=2^-10  DoSatur=off
  Saturation Dynamic1 : simulink/Discontinuities/Saturation Dynamic  OutMin=[]  OutMax=[]  OutDataTypeStr=Inherit: Same as second input  OutDataType=fixdt(1, 16)  OutScaling=2^-10  DoSatur=off
  Saturation1 : Saturate  UpperLimit=0  LowerLimit=-0.08
  Scope : Scope  Commented=on  NumInputPorts=2
  Scope1 : Scope  NumInputPorts=3
  Scope10 : Scope  Commented=on  NumInputPorts=4
  Scope11 : Scope  Commented=on  NumInputPorts=2
  Scope{2,4,6,9,13} (5 alike) : Scope  NumInputPorts=2
  Scope15 : Scope  Commented=on
  Scope16 : Scope  Commented=on  NumInputPorts=3
  Scope3 : Scope  Commented=on  NumInputPorts=2
  Scope5 : Scope  NumInputPorts=4
  Scope7 : Scope  Commented=on  NumInputPorts=4
  Scope8 : Scope  Commented=on  NumInputPorts=4
  Second-Order Filter1 : powerlib_meascontrol/Filters/Second-Order Filter  FilterType=Lowpass  Fo=Freq_filter  Zeta=Zeta_filter  Ts=Ts  Initialize=off  Vac_Init="[0,  0,  60]"  Vdc_Init=0  PlotResponse=off  FreqRange=[0, 500, 1]
      settings: SourceProductBaseCode=MT,PS
  Sqrt1 : Sqrt  SaturateOnIntegerOverflow=on
  Sqrt2 : Sqrt  SaturateOnIntegerOverflow=on
  Subtract : Sum  Inputs=+-
  Subtract1 : Sum  Inputs=+-
  Sum10 : Sum  Inputs=|+-
  Sum11 : Sum  Inputs=|-+
  Sum12 : Sum  Inputs=+-|
  Sum13 : Sum  Inputs=|+-
  Sum14 : Sum  Inputs=-+|
  Sum15 : Sum  Inputs=|+-
  Sum16 : Sum  Inputs=|++
  Sum3 : Sum  Inputs=|+-  InputSameDT=on  SaturateOnIntegerOverflow=on  OutDataTypeStr=Inherit: Same as first input
  Sum4 : Sum  Inputs=-+|  InputSameDT=on  SaturateOnIntegerOverflow=on  OutDataTypeStr=Inherit: Same as first input
  Sum6 : Sum  Inputs=||++-  InputSameDT=on  SaturateOnIntegerOverflow=on  OutDataTypeStr=Inherit: Same as first input
  Sum7 : Sum  Inputs=|+-  InputSameDT=on  SaturateOnIntegerOverflow=on  OutDataTypeStr=Inherit: Same as first input
  Sum8 : Sum  Inputs=|--+  InputSameDT=on  SaturateOnIntegerOverflow=on  OutDataTypeStr=Inherit: Same as first input
  Sum9 : Sum  Inputs=|-+  InputSameDT=on  SaturateOnIntegerOverflow=on  OutDataTypeStr=Inherit: Same as first input
  Switch : Switch  Criteria=u2 > Threshold  Threshold=2.5
  Switch Case : SwitchCase  CaseConditions={2, 3}
  Switch Case Action Subsystem : Subsystem  TreatAsAtomicUnit=on
  Switch Case Action Subsystem1 : Subsystem  TreatAsAtomicUnit=on
  Switch Case Action Subsystem2 : Subsystem  TreatAsAtomicUnit=on
  Switch Case Action Subsystem3 : Subsystem  TreatAsAtomicUnit=on
  Switch Case1 : SwitchCase  CaseConditions={2, 3}
  Switch{1..3,5} (4 alike) : Switch  Criteria=u2 > Threshold
  Switch7 : Switch  Commented=on  Criteria=u2 > Threshold  Threshold=0.5
  V0 : Constant  Value=0
  avoid neg i : Saturate  UpperLimit=i_max^2  LowerLimit=0
  avoid neg r : Saturate  UpperLimit=i_max^2  LowerLimit=0
  dq0 to abc : powerlib_meascontrol/Transformations/dq0 to abc  Alignment=90 degrees behind phase A axis
      settings: SourceProductBaseCode=MT,PS
  k_uvrt1 : Gain  Gain=k_uvrt
  k_uvrt2 : Gain  Gain=k_ovrt
  max 1 : Saturate  UpperLimit=1  LowerLimit=0
  open breaker : Logic  Operator=NOR  AllPortsSameDT=off  OutDataTypeStr=boolean
  "pu -> A1" : Gain  Gain=i_rated
  "pu -> A2" : Gain  Gain=i_rated
  protection : Outport
  Uctrl_inverter : Outport  Port=2  VectorParamsAs1DForOutWhenUnconnected=off
  wires:
  Logical Operator5/1 -> Product6/1
  [UVRT] -> Scope7/3, Logical Operator5/2
  [FRT_Mode1] -> Scope7/1, Logical Operator5/1
  Q_ref/1 -> Discrete Transfer Fcn1/1, Discrete Transfer Fcn1/2
  Discrete Transfer Fcn1/1 -> [Q_ref_filt]
  Product7/1 -> Add1/2
  "pu -> A2"/1 -> Product7/1
  Logical Operator6/1 -> Product7/2
  [FRT_Mode1] -> Logical Operator6/2
  [OVRT] -> Scope7/2, Logical Operator6/1
  Sum12/1 -> Saturation1/1
  k_uvrt2/1 -> "pu -> A2"/1
  Compare To Constant6/1 -> [FRT_Mode2]
  Compare To Constant5/1 -> [FRT_Mode1]
  [u_frt] -> Sum12/2
  Constant12/1 -> Sum12/1
  Add1/1 -> Scope7/4, Discrete Transfer Fcn3/1
  Product6/1 -> Add1/1
  "pu -> A1"/1 -> Product6/2
  Sum11/1 -> Saturation/1
  k_uvrt1/1 -> "pu -> A1"/1
  [u_frt] -> Scope13/1, Sum11/1
  Constant9/1 -> Scope13/2, Sum11/2
  Vdc_meas/1 -> Discrete Transfer Fcn2/1, Scope/1, [Vdc_meas]
  Discrete Transfer Fcn2/1 -> Scope/2, [Vdc_filt]  "Vdc_filt"
  Subtract/1 -> [u_frt], Switch Case Action Subsystem1/1(u_frt), Switch Case Action Subsystem/1(u_frt)  "u_Frt"
  Avoid FRT during initialization/1 -> AND/1
  avoid neg r/1 -> Sqrt1/1
  avoid neg i/1 -> Sqrt2/1
  [i_q] -> Math Function3/1
  [reac_prio] -> Scope10/3, Switch2/2
  Sqrt2/1 -> Scope10/2, Switch2/3
  Constant18/1 -> Scope10/1, Switch2/1
  [reac_prio] -> Scope15/1, Switch1/2
  Constant16/1 -> Switch1/3
  Sqrt1/1 -> Switch1/1
  [i_d] -> Math Function5/1
  Sum14/1 -> avoid neg i/1
  Constant11/1 -> Math Function4/1
  Sum13/1 -> avoid neg r/1
  Math Function3/1 -> Sum13/2
  Math Function2/1 -> Sum13/1
  Constant6/1 -> Math Function2/1
  Math Function4/1 -> Sum14/2
  Math Function5/1 -> Sum14/1
  Switch1/1 -> Switch3/3, Scope16/3
  Switch3/1 -> Delay/1
  [id0_FRT2] -> Scope16/1, Switch3/1
  [reset_id_FRT2] -> Scope16/2, Switch3/2
  Switch2/1 -> Switch5/3
  [iq0_FRT2] -> Abs4/1
  [reset_iq_FRT2] -> Scope10/4, Switch5/2
  Switch5/1 -> Delay1/1
  Delay/1 -> Scope2/1, [i_d_lim]
  Delay1/1 -> Scope2/2, [i_q_lim]
  Constant2/1 -> PI with anti-windup and dynamic limits - Id/3(LowerLimit)
  [i_q_lim] -> Gain1/1
  [i_q_lim] -> Saturation Dynamic1/1
  Gain1/1 -> Saturation Dynamic1/3
  [i_d_lim] -> Saturation Dynamic/1
  Saturation Dynamic1/1 -> Delay3/1
  Saturation Dynamic/1 -> Delay2/1
  Constant4/1 -> Saturation Dynamic/3
  PQ_meas/1 -> Demux2/1
  [i_d_lim] -> Mux4/1, PI with anti-windup and dynamic limits - Id/1(UpperLimit)  "i_d_lim"
  Demux2/2 -> Discrete Transfer Fcn4/1
  Abs4/1 -> Switch5/1
  [FRT_flag] -> Compare To Constant/1
  Discrete-Time Integrator2/1 -> Switch Case Action Subsystem2/1(u_frt), Switch Case Action Subsystem3/1(u_frt)
  Data Type Conversion4/1 -> Discrete-Time Integrator2/2, Discrete-Time Integrator2/1
  Merge2/1 -> Counter AST/Trigger
  Counter AST/1(Count) -> max 1/1
  Compare To Constant/1 -> Data Type Conversion4/1
  max 1/1 -> Scope4/1, open breaker/1
  u_f_protect/1 -> open breaker/2
  open breaker/1 -> protection/1, Scope4/2, [protection]
  [FRT_Mode2] -> Logical Operator4/1
  [FRT_flag] -> Logical Operator4/2
  [i_d] -> Delay d1/1
  [i_q] -> Delay q1/1
  Delay d1/1 -> Sample and Hold d1/1, Sample and Hold d/1
  Delay q1/1 -> Sample and Hold q/1
  Edge Detector1/1 -> Sample and Hold d/2, Sample and Hold q/2
  Constant13/1 -> Discrete-Time Integrator3/1
  Discrete-Time Integrator3/1 -> Compare To Constant7/1
  Compare To Constant7/1 -> Data Type Conversion1/1
  Product5/1 -> Predictor1/1(in)
  Product8/1 -> Predictor2/1(in)
  Sample and Hold q/1 -> Product8/1
  Predictor2/1(out) -> Scope8/3, [iq0_FRT2]  "iq0"
  FRT_ramp_q/1(y) -> Compare To Constant9/1, Product8/2
  Compare To Constant9/1 -> Scope8/4, [reset_iq_FRT2]  "reset iq"
  FRT_ramp_p/1(y) -> Compare To Constant8/1, Product5/2
  [Vdc_filt] -> Relay3/1
  Compare To Constant8/1 -> Logical Operator11/1
  Logical Operator11/1 -> Logical Operator1/1
  Logical Operator4/1 -> Discrete-Time Integrator3/2, Logical Operator1/2, Edge Detector1/1
  Logical Operator1/1 -> Scope8/2, [reset_id_FRT2]  "reset id"
  Data Type Conversion1/1 -> FRT_ramp_q/2(u), FRT_ramp_p/2(u)
  Relay3/1 -> Logical Operator11/2
  Constant19/1 -> FRT_ramp_p/1(UpperLimit)
  Constant20/1 -> FRT_ramp_p/3(LowerLimit)
  Constant22/1 -> FRT_ramp_q/1(UpperLimit)
  Constant23/1 -> FRT_ramp_q/3(LowerLimit)
  Switch/1 -> PI with anti-windup and dynamic limits - Id/5(x_reset)
  [FRT_Mode1] -> Logical Operator3/1
  [FRT_flag] -> Logical Operator3/2
  Logical Operator3/1 -> Edge Detector4/1, Edge Detector3/1, [reac_prio]
  Edge Detector3/1 -> Sample and Hold d1/2
  Sample and Hold d1/1 -> [id0_FRT1], Scope11/1
  Edge Detector4/1 -> Data Type Conversion2/1
  Data Type Conversion2/1 -> Scope11/2, [reset_id_FRT1]
  [reset_id_FRT1] -> Logical Operator7/1, Scope9/1
  [reset_id_FRT2] -> Scope9/2, Logical Operator7/2
  Logical Operator7/1 -> PI with anti-windup and dynamic limits - Id/4(Reset)
  [mode] -> Switch/2
  [id0_FRT1] -> Switch/3
  [id0_FRT2] -> Switch/1
  Predictor1/1(out) -> Scope8/1, [id0_FRT2]  "id0"
  Delay2/1 -> Product1/1
  Delay3/1 -> Product2/2
  [protection] -> Product2/1, Product1/2
  Product2/1 -> Gain/1
  Product4/1 -> PI with anti-windup and dynamic limits - Id/2(Input)
  [protection] -> Product4/1
  [i_d] -> Saturation Dynamic/2
  [i_q] -> Saturation Dynamic1/2
  Sample and Hold d/1 -> Product5/1
  Logical Operator2/1 -> Avoid FRT during initialization/1
  Constant3/1 -> Avoid FRT during initialization/3
  Digital Clock2/1 -> Avoid FRT during initialization/2
  [Vdc_meas] -> Avoid division by zero/1
  Cartesian to Polar/1 -> Product13/1
  Product13/1 -> 0-Mod_index_max/1  "m"
  Demux4/1 -> [Vd]
  w_pu/1 -> [w_pu]
  [iq_ref] -> Product/3
  Sum7/1 -> Mux2/1
  [w_pu] -> Product/2
  Product11/1 -> Sum6/3
  Avoid division by zero/1 -> Product13/3
  Product12/1 -> Sum8/1
  Demux3/2 -> Sum9/1  "vq'"
  Constant10/1 -> Product11/1
  Discrete PI Controller1/1(Out) -> Demux3/1
  Mux2/1 -> Discrete PI Controller1/1(Error)
  Product/1 -> Sum6/2
  Product1/1 -> Gain2/1
  Vdq_grid/1 -> Demux4/1
  Gain/1 -> Sum4/2, [iq_ref], Scope5/4
  Demux3/1 -> Sum3/2  "vd'"
  Constant8/1 -> Product10/2
  Product10/1 -> Sum8/2
  [Vd] -> Sum6/1
  Constant17/1 -> Product12/2
  [w_pu] -> Product10/3
  Sum8/1 -> Sum9/2
  Demux/1 -> Sum7/2, Scope5/1, [id]  "id"
  [id_ref] -> Product10/1
  dq0 to abc/1 -> Uctrl_inverter/1  "Uctrl"
  Polar to Cartesian/2 -> Mux/2
  Sum6/1 -> Sum3/1
  K/1 -> Product13/2
  Mux/1 -> dq0 to abc/1  "Vdq0"
  [Vq] -> Sum8/3
  Sum3/1 -> Cartesian to Polar/1  "Vd inverter"
  [iq_ref] -> Product12/1
  Cartesian to Polar/2 -> Polar to Cartesian/2  "Phase"
  0-Mod_index_max/1 -> Polar to Cartesian/1
  Sum9/1 -> Cartesian to Polar/2  "Vq inverter"
  [id_ref] -> Product11/2
  Constant5/1 -> Product/1
  Polar to Cartesian/1 -> Mux/1
  Sum4/1 -> Mux2/2
  Demux4/2 -> [Vq]
  V0/1 -> Mux/3
  Theta_PLL/1 -> dq0 to abc/2
  Idq_gc/1 -> Demux/1
  PI with anti-windup and dynamic limits - Id/1(Output) -> [i_d], Mux4/2  "i_d_ref"
  Gain2/1 -> Scope5/2, Sum7/1, [id_ref]
  ->pu/1 -> Product4/2  "Vdc_filt"
  Constant21/1 -> Sum10/2
  [Vdc_filt] -> Sum10/1
  Mux4/1 -> Scope3/1
  Mux3/1 -> Scope3/2
  Demux/2 -> Scope5/3, Sum4/1, [iq]  "iq"
  [id] -> Gain7/1
  Gain9/1 -> Mux3/3  "iq"
  Gain7/1 -> Mux4/3  "id"
  [iq] -> Gain9/1  "iq"
  [iq0_FRT2] -> PI with anti-windup and dynamic limits - Iq/5(x_reset)
  [FRT_flag] -> Logical Operator9/1
  [i_q_lim] -> Mux3/1, PI with anti-windup and dynamic limits - Iq/1(UpperLimit)
  PI with anti-windup and dynamic limits - Iq/1(Output) -> Scope6/2, Sum16/1
  Product14/1 -> Product15/2
  [Q_ref_filt] -> Sum15/1
  [reset_iq_FRT2] -> PI with anti-windup and dynamic limits - Iq/4(Reset)
  Logical Operator9/1 -> Product14/2
  Sum15/1 -> Gain5/1
  Sum16/1 -> Mux3/2, [i_q]  "iq"
  [Q_meas_filt] -> Sum15/2
  [i_q_lim] -> Gain10/1
  [di_imag_uvrt] -> Scope6/1, Sum16/2
  Product15/1 -> PI with anti-windup and dynamic limits - Iq/2(Input)
  [protection] -> Product15/1
  Gain10/1 -> PI with anti-windup and dynamic limits - Iq/3(LowerLimit)
  Saturation/1 -> k_uvrt1/1
  Saturation1/1 -> k_uvrt2/1
  Discrete Transfer Fcn3/1 -> [di_imag_uvrt]  "Vdc_filt"
  Sum10/1 -> ->pu/1  "Vdc_filt"
  Gain5/1 -> Product14/1
  Discrete Transfer Fcn4/1 -> Second-Order Filter1/1
  Second-Order Filter1/1 -> [Q_meas_filt]
  AND/1 -> Scope1/3, [FRT_flag]
  Digital Clock3/1 -> Less Than2/1, GreaterThan2/1
  Constant28/1 -> Less Than2/2
  Constant27/1 -> GreaterThan2/2
  From7/1 -> Switch7/1  "i_d_lim"
  AND3/1 -> Switch7/2
  GreaterThan2/1 -> AND3/2
  Less Than2/1 -> AND3/1
  [mode] -> Switch Case/1
  Merge/1 -> Scope1/1, Logical Operator2/1, [OVRT]
  Switch Case Action Subsystem/1(Out1) -> Merge/1
  Switch Case Action Subsystem1/1(Out1) -> Merge/2
  Switch Case Action Subsystem/2(Output) -> Merge1/1
  Switch Case Action Subsystem1/2(Output) -> Merge1/2
  Merge1/1 -> Scope1/2, [UVRT], Logical Operator2/2
  [mode] -> Switch Case1/1
  Switch Case Action Subsystem2/1(Out1) -> Merge2/1
  Switch Case Action Subsystem3/1(Out1) -> Merge2/2
  u_frt/1 -> Subtract/1  "u_Frt"
  V_Setpoint/1 -> Subtract1/1
  Subtract1/1 -> Subtract/2  "u_Frt"
  Constant/1 -> Subtract1/2
  OR/1 -> AND/2
  Mode/1 -> [mode], Compare To Constant6/1, Compare To Constant5/1
  [FRT_Mode1] -> OR/1
  [FRT_Mode2] -> OR/2
  Switch Case1/1 -> Switch Case Action Subsystem2/Action
  Switch Case1/2 -> Switch Case Action Subsystem3/Action
  Switch Case/1 -> Switch Case Action Subsystem/Action
  Switch Case/2 -> Switch Case Action Subsystem1/Action
